simulink model "LED_Cmd_varZ_expResults"  (Simulink 7.8)
settings: Solver=FixedStepDiscrete  StartTime=0.0  StopTime=10.0  RelTol=1e-3  SampleTimeConstraint=STIndependent
PreLoadFcn:
  | LED_Cmd_varZ_selfinit
CloseFcn:
  | rtwprivate ssgencode ModelCloseRequest ADL
settings Model: MinMaxOverflowLogging=ForceOff  SldvGeneratedHarnessModel=TestUnitModel=LED_Cmd_varZ|  Creator=fguerin  LastModifiedBy=klindqvi  CovMetricSettings=dcmoe  CovHTMLOptions=-aTS=1 -bRG=1 -bTC=0 -hTR=0 -nFC=0 -scm=1 -bcm=1  covSaveCumulativeToWorkspaceVar=off  CovSaveSingleToWorkspaceVar=off  CovModelRefEnable=on  CovExternalEMLEnable=on
settings DataIOCC: LimitDataPoints=off  SaveFormat=StructureWithTime  SaveOutput=off  SignalLogging=off  DSMLogging=off  SaveTime=off  SignalLoggingName=logsOut
settings OptimizationCC: InlineParams=on  InlineInvariantSignals=on  EnhancedBackFolding=on  PassReuseOutputArgsAs=Individual arguments  ZeroExternalMemoryAtStartup=off  ZeroInternalMemoryAtStartup=off  EfficientFloat2IntCast=on  OptimizeModelRefInitCode=on
settings DebuggingCC: SignalInfNanChecking=error  SignalRangeChecking=error  ReadBeforeWriteMsg=EnableAllAsError  WriteAfterWriteMsg=EnableAllAsError  WriteAfterReadMsg=EnableAllAsError  AlgebraicLoopMsg=error  ArtificialAlgebraicLoopMsg=error  SaveWithDisabledLinksMsg=error  SaveWithParameterizedLinksMsg=error  CheckExecutionContextPreStartOutputMsg=on  CheckExecutionContextRuntimeOutputMsg=on  BlockPriorityViolationMsg=error  SolverPrmCheckMsg=error  InheritedTsInSrcMsg=none  MultiTaskCondExecSysMsg=warning  MultiTaskRateTransMsg=warning  CheckMatrixSingularityMsg=error  IntegerOverflowMsg=error  ParameterUnderflowMsg=error  ParameterPrecisionLossMsg=error  ParameterTunabilityLossMsg=error  UnderSpecifiedDataTypeMsg=warning  UnnecessaryDatatypeConvMsg=warning  VectorMatrixConversionMsg=error  SignalLabelMismatchMsg=warning  SFcnCompatibilityMsg=error  BusObjectLabelMismatch=error  RootOutportRequireBusObject=error  AssertControl=DisableAll  ModelReferenceIOMsg=error  ModelReferenceIOMismatchMessage=error  ModelReferenceCSMismatchMessage=warning  UnknownTsInhSupMsg=error  ModelReferenceDataLoggingMessage=error  StrictBusMsg=ErrorOnBusTreatedAsVector
settings HardwareCC: ProdLargestAtomicInteger=Long  ProdLargestAtomicFloat=Double  ProdIntDivRoundTo=Zero  ProdEndianess=BigEndian  ProdHWDeviceType=Freescale->MPC5500
settings ModelReferenceCC: ModelReferenceNumInstancesAllowed=Single
settings SFSimCC: SimParseCustomCode=off
settings RTWCC: SystemTargetFile=autosar.tlc  TemplateMakefile=ert_default_tmf  Description=AUTOSAR  GenerateReport=on  ProcessScript=autosar_make_rtw_hook  IncludeHyperlinkInReport=on  LaunchReport=on  GenerateTraceInfo=on  GenerateTraceReport=on  GenerateTraceReportSl=on  GenerateTraceReportSf=on  GenerateTraceReportEml=on
settings CodeAppCC: ForceParamTrailComments=on  IgnoreCustomStorageClasses=off  IgnoreTestpoints=on  MangleLength=4  InlinedPrmAccess=Macros  ReqsInCode=on
settings STFCustomTargetCC: UtilityFuncGeneration=Shared location  ParMdlRefBuildCompliant=on  CompOptLevelCompliant=on  IncludeMdlTerminateFcn=off  GeneratePreprocessorConditionals=Use local settings  CombineOutputUpdateFcns=on  SuppressErrorStatus=on  ERTFirstTimeCompliant=on  ERTCustomFileBanners=on  SupportNonFinite=off  SupportComplex=off  SupportContinuousTime=off  SupportNonInlinedSFcns=off  PortableWordSizes=on  AutosarCompliant=on  SystemTargetFile=autosar.tlc
settings ERTTargetCC: UtilityFuncGeneration=Shared location  MultiwordLength=2048  ConcurrentExecutionCompliant=off  IncludeMdlTerminateFcn=off  SuppressErrorStatus=on  SupportNonFinite=off  SupportComplex=off  PortableWordSizes=on  ModelStepFunctionPrototypeControlCompliant=off  CPPClassGenCompliant=off  AutosarCompliant=on  GenerateErtSFunction=on  CreateSILPILBlock=SIL  GenerateASAP2=on  ExtModeMexFile=noextcomm  InlinedParameterPlacement=NonHierarchical  ERTCustomFileTemplate=example_file_process.tlc  ERTFilePackagingFormat=Compact  ConvertIfToSwitch=off  SuppressUnreachableDefaultCases=off
settings CustomProperty: DataType=RTWOptions_EnumType__toolbox_rtw_targets_autosar_autosar_autosar_1_1AutosarSchemaVersion  Value=3.0
settings EnumStrPairs: String=2.0
settings ConfigComp: Description=Design Verifier Custom Configuration Component  DVMaxProcessTime=600  DVDisplayUnsatisfiableObjectives=on  DVAutomaticStubbing=off  DVModelCoverageObjectives=MCDC  DVTestSuiteOptimization=CombinedObjectives  DVDataFileName=./Tests/LED_Cmd_varZ_sldvdata  DVSaveHarnessModel=on  DVHarnessModelFileName=LED_Cmd_varZ_testHarness  DVSaveReport=on  DVReportFileName=ADL_Sim_SLDV.html

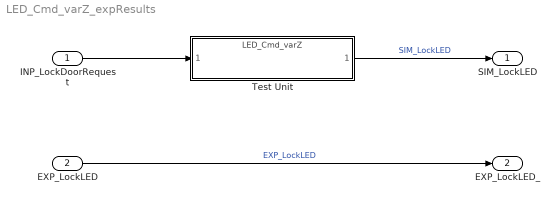
== system LED_Cmd_varZ_expResults ==
  INP_LockDoorRequest : Inport
  EXP_LockLED : Inport  Port=2
  Test Unit : ModelReference  ModelNameDialog=LED_Cmd_varZ  SimulationMode=Normal  ModelReferenceVersion=1.319  CopyOfModelName=LED_Cmd_varZ  DefaultDataLogging=off
  SIM_LockLED : Outport
  EXP_LockLED_ : Outport  Port=2
  wires:
  INP_LockDoorRequest/1 -> Test Unit/1
  Test Unit/1 -> SIM_LockLED/1  "SIM_LockLED"
  EXP_LockLED/1 -> EXP_LockLED_/1  "EXP_LockLED"
